simulink model "buckwtih_RCsnubber"  (R2017b)
settings: Solver=VariableStepAuto  StartTime=0.0  StopTime=1  FixedStep=1e-6  MaxStep=1e-4  RelTol=1e-3
libraries: powerlib x16, powerlib_meascontrol x1, simulink x1
settings Model: Creator=anılcanbudak  LastModifiedBy=SiF

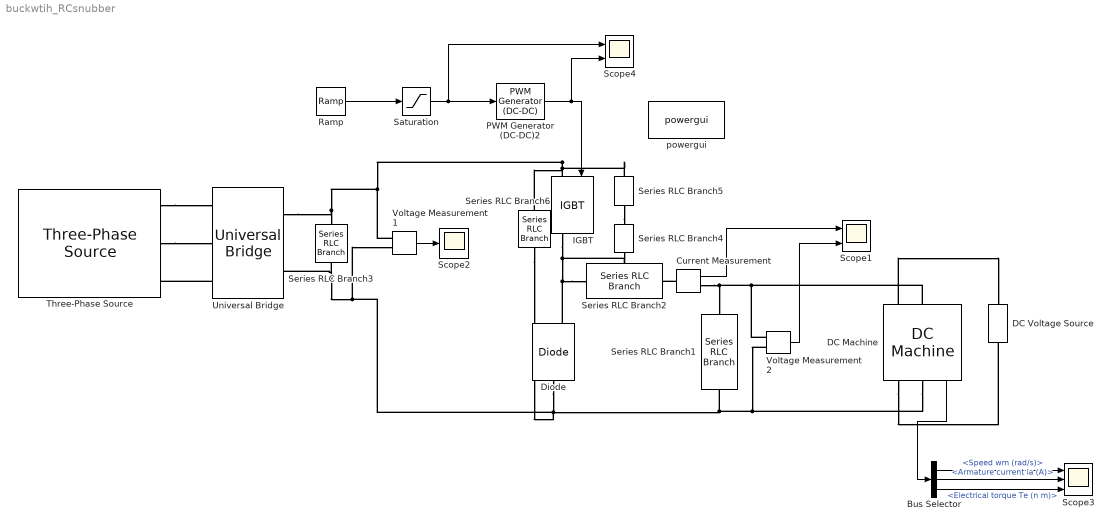
== system buckwtih_RCsnubber ==
  Bus Selector : BusSelector  OutputSignals=Speed wm (rad/s),Armature current ia (A),Electrical torque Te (n m)
  Current Measurement : powerlib/Measurements/Current Measurement  PhasorSimulation=off  OutputType=Complex  PSBequivalent=0
  DC Machine : powerlib/Machines/DC Machine  PresetModel=No  MechanicalLoad=Torque TL  FieldType=Wound  ShowDetailedParameters=on  MeasurementBus=off  RLa="[ 0.6  0.012]"  RLf="[ 240  120]"  Laf=1.5  MachineConstant=Torque constant (N.m/A)  Ke=1.8  Kt=1.8  J=1  Bm=0  Tf=0  w0=1  Ifinit=1  TsPowergui=0  TsBlock=-1
  DC Voltage Source : powerlib/Electrical Sources/DC Voltage Source  Amplitude=220  Measurements=None
  Diode : powerlib/Power Electronics/Diode  Ron=0  Lon=0  Vf=0  IC=0  UseSnubber=0  Rs=500  Cs=250e-9  Measurements=on
  IGBT : powerlib/Power Electronics/IGBT  Ron=0  Lon=0  Vf=0  Tf=1e-6  Tt=2e-6  IC=0  Rs=1e5  Cs=inf  Measurements=on
  PWM Generator (DC-DC)2 : powerlib_meascontrol/Pulse & Signal Generators/PWM Generator (DC-DC)  Fsw=500  Ts=0
  Ramp : simulink/Sources/Ramp  slope=2  start=0  X0=0
  Saturation : Saturate  UpperLimit=0.95  LowerLimit=-1
  Scope1 : Scope  NumInputPorts=2
  Scope2 : Scope
  Scope3 : Scope  NumInputPorts=3
  Scope4 : Scope  NumInputPorts=2
  Series RLC Branch1 : powerlib/Elements/Series RLC Branch  LConnTagsString=__new0  RConnTagsString=__new0  BranchType=C  Resistance=1  Inductance=1e-3  SetiL0=off  InitialCurrent=0  Capacitance=660e-6  Setx0=off  InitialVoltage=0  Measurements=None
  Series RLC Branch2 : powerlib/Elements/Series RLC Branch  LConnTagsString=__new0  RConnTagsString=__new0  BranchType=L  Resistance=1  Inductance=4e-3  SetiL0=off  InitialCurrent=0  Capacitance=1e-6  Setx0=off  InitialVoltage=0  Measurements=None
  Series RLC Branch3 : powerlib/Elements/Series RLC Branch  LConnTagsString=__new0  RConnTagsString=__new0  BranchType=C  Resistance=1  Inductance=1e-3  SetiL0=off  InitialCurrent=0  Capacitance=680e-6  Setx0=off  InitialVoltage=0  Measurements=None
  Series RLC Branch4 : powerlib/Elements/Series RLC Branch  LConnTagsString=__new0  RConnTagsString=__new0  BranchType=C  Resistance=1  Inductance=1e-3  SetiL0=off  InitialCurrent=0  Capacitance=9e-9  Setx0=off  InitialVoltage=0  Measurements=None
  Series RLC Branch5 : powerlib/Elements/Series RLC Branch  LConnTagsString=__new0  RConnTagsString=__new0  BranchType=R  Resistance=100  Inductance=1e-3  SetiL0=off  InitialCurrent=0  Capacitance=1e-3  Setx0=off  InitialVoltage=0  Measurements=None
  Series RLC Branch6 : powerlib/Elements/Series RLC Branch  LConnTagsString=__new0  RConnTagsString=__new0  BranchType=C  Resistance=1  Inductance=1e-3  SetiL0=off  InitialCurrent=0  Capacitance=1e-6  Setx0=off  InitialVoltage=0  Measurements=None
  Three-Phase Source : powerlib/Electrical Sources/Three-Phase Source  InternalConnection=Yg  VoltagePhases=off  Voltage=170  PhaseAngle=0  Voltage_phases=[25e3 25e3 25e3]/sqrt(3)  PhaseAngles_phases=[0 -120 +120]  Frequency=50  NonIdealSource=on  SpecifyImpedance=off  Resistance=0.1  Inductance=100e-06  ShortCircuitLevel=100e6  BaseVoltage=170  XRratio=7  BusType=swing  Pref=10e3  Qref=0  Prefabc=[10e3, 10e3, 10e3]  Qrefabc=[0, 0, 0]  Qmin=-inf  Qmax=inf
  Universal Bridge : powerlib/Power Electronics/Universal Bridge  Arms=3  SnubberResistance=1e5  SnubberCapacitance=inf  Device=Diodes  Ron=1e-3  Lon=0  ForwardVoltages="[  0  0  ]"  ForwardVoltage=0  GTOparameters=[ 10e-6 , 20e-6 ]  IGBTparameters=[ 1e-6 , 2e-6 ]  Measurements=None  Measurements_2=None  converterType=Rectifier
  Voltage Measurement1 : powerlib/Measurements/Voltage Measurement  PhasorSimulation=off  OutputType=Complex  PSBequivalent=0
  Voltage Measurement2 : powerlib/Measurements/Voltage Measurement  PhasorSimulation=off  OutputType=Complex  PSBequivalent=0
  powergui : powerlib/powergui  Priority=1  SimulationMode=Continuous  SampleTime=50e-6  frequency=60  Iterations=50  frequencyindice=0  Pbase=100e6  ErrMax=1e-4  UnitsV=kV  UnitsW=MW  buscounter=0  FunctionMessages=off  echomessages=off  EnableUseOfTLC=off  CurrentSourceSwitches=off  DisableSnubberDevices=off  DisableRonSwitches=off  DisableVfSwitches=off  DisplayEquations=off  SolverType=Tustin/Backward Euler (TBE)  Interpol=off  ExternalGateDelay=off  methode=off  Ts=100  x0status=blocks  SPID=on  SwTol=0  HookPort=off  RestoreLinks=warning  ResistiveCurrentMeasurement=off  Frange=[0:2:500]  Ylog=off  Xlog=on  ShowGrid=off  save=off  variable=ZData  structure=0  ZoomFFT=off  StartTime=0.0  cycles=1  DisplayStyle=1  fundamental=60  FreqAxis=off  MaxFrequency=1000  frequencyindicesteady=1  RmsSteady=1  display=off
  wires:
  Current Measurement/1 -> Scope1/1
  Saturation/1 -> Scope4/1, PWM Generator (DC-DC)2/1
  PWM Generator (DC-DC)2/1 -> Scope4/2, IGBT/1
  Voltage Measurement1/1 -> Scope2/1
  DC Machine/1 -> Bus Selector/1
  Bus Selector/1 -> Scope3/1  "<Speed wm (rad/s)>"
  Bus Selector/2 -> Scope3/2  "<Armature current ia (A)>"
  Bus Selector/3 -> Scope3/3  "<Electrical torque Te (n m)>"
  Voltage Measurement2/1 -> Scope1/2
  Ramp/1 -> Saturation/1
  connections:
  Series RLC Branch6/RConn1 -- Diode/LConn1 -- Universal Bridge/RConn2 -- Series RLC Branch3/RConn1 -- Voltage Measurement1/LConn2 -- Voltage Measurement2/LConn2 -- DC Machine/RConn1 -- Series RLC Branch1/RConn1
  Current Measurement/RConn1 -- DC Machine/LConn1 -- Voltage Measurement2/LConn1 -- Series RLC Branch1/LConn1
  Series RLC Branch3/LConn1 -- Series RLC Branch5/LConn1 -- Series RLC Branch6/LConn1 -- IGBT/LConn1 -- Voltage Measurement1/LConn1 -- Universal Bridge/RConn1
  Series RLC Branch2/LConn1 -- Diode/RConn1 -- Series RLC Branch4/RConn1 -- IGBT/RConn1
  Three-Phase Source/RConn1 -- Universal Bridge/LConn1
  Three-Phase Source/RConn2 -- Universal Bridge/LConn2
  Universal Bridge/LConn3 -- Three-Phase Source/RConn3
  Current Measurement/LConn1 -- Series RLC Branch2/RConn1
  DC Machine/LConn2 -- DC Voltage Source/RConn1
  DC Machine/RConn2 -- DC Voltage Source/LConn1
  Series RLC Branch5/RConn1 -- Series RLC Branch4/LConn1
